simulink model "KiemChungDynamic"  (R2022a)
settings: Solver=FixedStepAuto  StartTime=0.0  StopTime=50  FixedStep=0.01  RelTol=1e-3
settings Model: Creator=Vũ Quốc Khánh  LastModifiedBy=Vũ Quốc Khánh

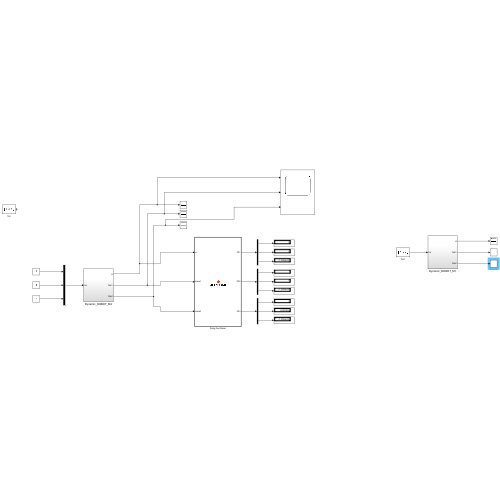
[thumbnail: Simulink's stored preview of the top-level diagram]
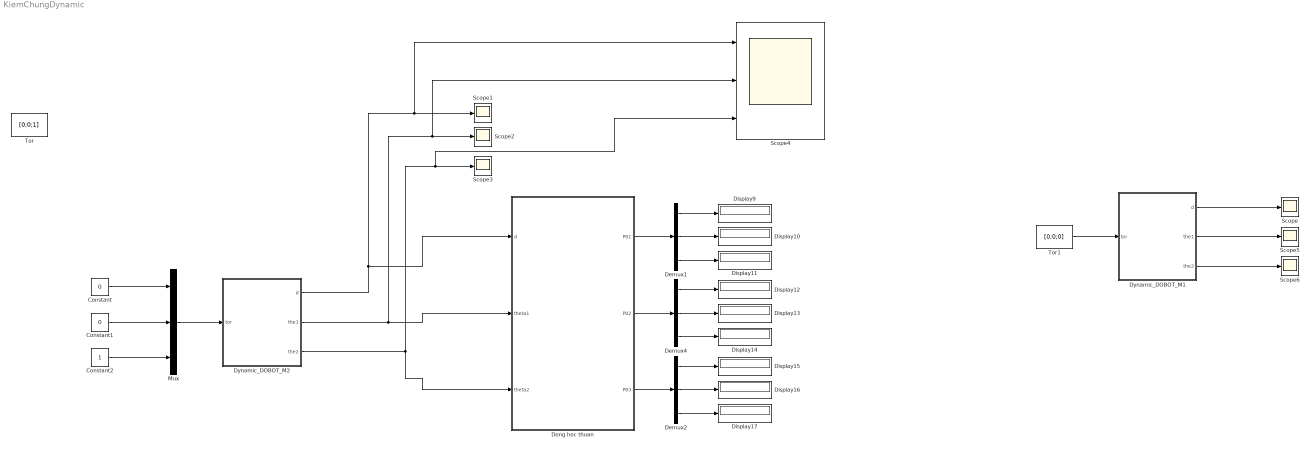
== system KiemChungDynamic ==
  Constant : Constant  Value=0
  Constant1 : Constant  Value=0
  Constant2 : Constant
  Demux1 : Demux  Outputs=3
  Demux2 : Demux  Outputs=3
  Demux4 : Demux  Outputs=3
  Display{9..17} (9 alike) : Display
  Dong hoc thuan : MATLAB Function  TreatAsAtomicUnit=on
  Dynamic_DOBOT_M1 : Subsystem
  Dynamic_DOBOT_M2 : Subsystem
  Mux : Mux  Inputs=3
  Scope{,1..3,5..6} (6 alike) : Scope
  Scope4 : Scope  NumInputPorts=3
  Tor : Constant  Value=[0;0;1]
  Tor1 : Constant  Value=[0;0;0]
  wires:
  Dynamic_DOBOT_M2/2(the1) -> Scope4/2, Scope2/1, Dong hoc thuan/2(theta1)
  Dynamic_DOBOT_M2/3(the2) -> Dong hoc thuan/3(theta2), Scope3/1, Scope4/3
  Dong hoc thuan/1(P01) -> Demux1/1
  Dong hoc thuan/2(P02) -> Demux4/1
  Dong hoc thuan/3(P03) -> Demux2/1
  Demux4/1 -> Display12/1
  Demux2/1 -> Display15/1
  Demux1/1 -> Display9/1
  Demux2/2 -> Display16/1
  Demux1/3 -> Display11/1
  Demux1/2 -> Display10/1
  Demux4/2 -> Display13/1
  Demux4/3 -> Display14/1
  Demux2/3 -> Display17/1
  Dynamic_DOBOT_M2/1(d) -> Scope4/1, Scope1/1, Dong hoc thuan/1(d)
  Constant/1 -> Mux/1
  Constant1/1 -> Mux/2
  Constant2/1 -> Mux/3
  Mux/1 -> Dynamic_DOBOT_M2/1(tor)
  Tor1/1 -> Dynamic_DOBOT_M1/1(tor)
  Dynamic_DOBOT_M1/2(the1) -> Scope5/1
  Dynamic_DOBOT_M1/3(the2) -> Scope6/1
  Dynamic_DOBOT_M1/1(d) -> Scope/1

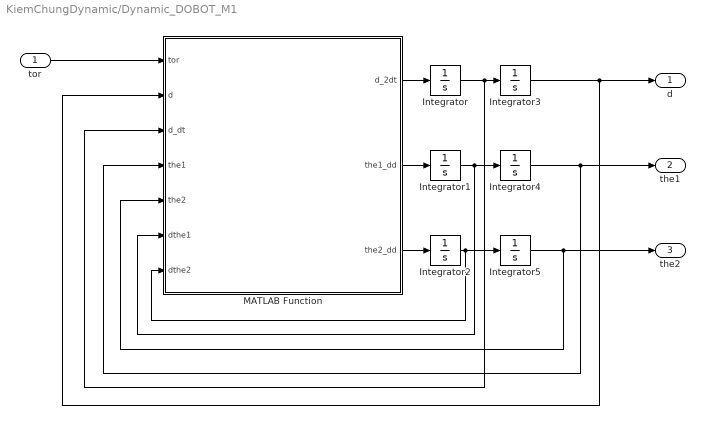
== system KiemChungDynamic/Dynamic_DOBOT_M1 ==
  tor : Inport
  Integrator{,1..5} (6 alike) : Integrator
  MATLAB Function : MATLAB Function  TreatAsAtomicUnit=on
  d : Outport  VectorParamsAs1DForOutWhenUnconnected=off
  the1 : Outport  Port=2  VectorParamsAs1DForOutWhenUnconnected=off
  the2 : Outport  Port=3  VectorParamsAs1DForOutWhenUnconnected=off
  wires:
  MATLAB Function/2(the1_dd) -> Integrator1/1
  Integrator4/1 -> MATLAB Function/4(the1), the1/1
  MATLAB Function/3(the2_dd) -> Integrator2/1
  Integrator/1 -> Integrator3/1, MATLAB Function/3(d_dt)
  Integrator3/1 -> MATLAB Function/2(d), d/1
  Integrator1/1 -> Integrator4/1, MATLAB Function/6(dthe1)
  Integrator2/1 -> Integrator5/1, MATLAB Function/7(dthe2)
  MATLAB Function/1(d_2dt) -> Integrator/1
  Integrator5/1 -> MATLAB Function/5(the2), the2/1
  tor/1 -> MATLAB Function/1(tor)

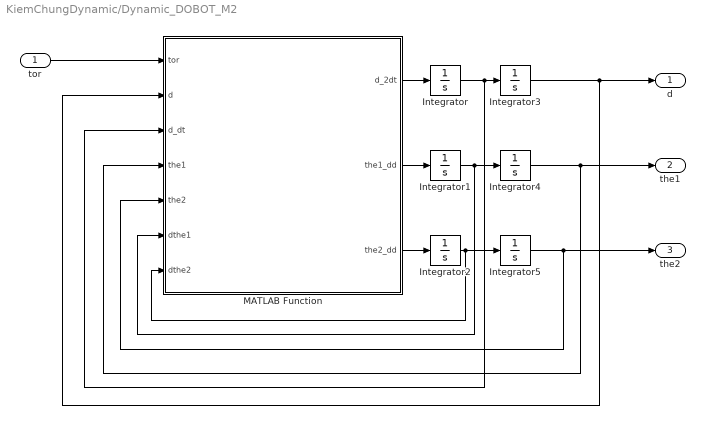
== system KiemChungDynamic/Dynamic_DOBOT_M2 ==
  tor : Inport
  Integrator{,1..5} (6 alike) : Integrator
  MATLAB Function : MATLAB Function  TreatAsAtomicUnit=on
  d : Outport  VectorParamsAs1DForOutWhenUnconnected=off
  the1 : Outport  Port=2  VectorParamsAs1DForOutWhenUnconnected=off
  the2 : Outport  Port=3  VectorParamsAs1DForOutWhenUnconnected=off
  wires:
  MATLAB Function/2(the1_dd) -> Integrator1/1
  Integrator4/1 -> MATLAB Function/4(the1), the1/1
  MATLAB Function/3(the2_dd) -> Integrator2/1
  Integrator/1 -> Integrator3/1, MATLAB Function/3(d_dt)
  Integrator3/1 -> MATLAB Function/2(d), d/1
  Integrator1/1 -> Integrator4/1, MATLAB Function/6(dthe1)
  Integrator2/1 -> Integrator5/1, MATLAB Function/7(dthe2)
  MATLAB Function/1(d_2dt) -> Integrator/1
  Integrator5/1 -> MATLAB Function/5(the2), the2/1
  tor/1 -> MATLAB Function/1(tor)

== matlab function KiemChungDynamic/Dong hoc thuan ==
  data: P01 output; P02 output; P03 output; d input; theta1 input; theta2 input
function [P01, P02, P03] = Dong_hoc_thuan(d,theta1, theta2)
L1=1; L2=1; L3=1;  %%cm
P01 = [0;0;d];
P02 = [L1;0;d];
P03 = [L1 + L2*cosd(theta1);
       L2*sind(theta1);
       d];
end

== matlab function KiemChungDynamic/Dynamic_DOBOT_M2/MATLAB Function ==
  data: tor input; d_2dt output; d input; d_dt input; the1 input; the2 input; dthe1 input; dthe2 input; the1_dd output; the2_dd output
function [d_2dt, the1_dd, the2_dd] = Dynamic(tor,d, d_dt,the1, the2, dthe1, dthe2)
m1=1; m2=1; m3=1;
L1=1; L2=1; L3=1;
g=9.81;
% MA Tran M
M11=m1+m2+m3;
M12=0;
M13=0;
M21=0;
M22=L2*L2*m2+L2*L2*m3+L3*L3*m3+2*L2*L3*m3*cos(the2);
M23=L3*m3*(L3+L2*cos(the2));
M31=0;
M32=L3*m3*(L3+L2*cos(the2));
M33=L3*L3*m3;
% Ma tran V
V11=0; 
V12= -L2*L3*dthe2*m3*sin(the2)*(2*dthe1+dthe2);
V13= L2*L3*the1*the1*m3*sin(the2);

% Ma tran G
G11=g*(m1+m2+m3);
G12=0;
G13=0;

M= [ M11,   M12,    M13;
     M21,   M22,    M23;
     M31,   M32,    M33;];
V=[V11; 
   V12;
   V13;];
G=[G11;
    G12;
    G13;];
the_dd=pinv(M)*(tor-G-V);
d_2dt=the_dd(1);
the1_dd=the_dd(2);
the2_dd=the_dd(3);
end

== matlab function KiemChungDynamic/Dynamic_DOBOT_M1/MATLAB Function ==
  data: tor input; d_2dt output; d input; d_dt input; the1 input; the2 input; dthe1 input; dthe2 input; the1_dd output; the2_dd output
function [d_2dt, the1_dd, the2_dd] = Dynamic(tor,d, d_dt,the1, the2, dthe1, dthe2)
m1=1; m2=1; m3=1;
L1=1; L2=1; L3=1;
g=9.81;
% MA Tran M
M11=m1+m2+m3;
M12=0;
M13=0;
M21=0;
M22=L2*L2*m2+L2*L2*m3+L3*L3*m3+2*L2*L3*m3*cos(the2);
M23=L3*m3*(L3+L2*cos(the2));
M31=0;
M32=L3*m3*(L3+L2*cos(the2));
M33=L3*L3*m3;
% Ma tran V
V11=0; 
V12= -L2*L3*dthe2*m3*sin(the2)*(2*dthe1+dthe2);
V13= L2*L3*the1*the1*m3*sin(the2);

% Ma tran G
G11=g*(m1+m2+m3);
G12=0;
G13=0;

M= [ M11,   M12,    M13;
     M21,   M22,    M23;
     M31,   M32,    M33;];
V=[V11; 
   V12;
   V13;];
G=[G11;
    G12;
    G13;];
the_dd=pinv(M)*(tor-G-V);
d_2dt=the_dd(1);
the1_dd=the_dd(2);
the2_dd=the_dd(3);
end
